simulink model "straight_forward_uniform_wind"  (R2020b)
settings: Solver=VariableStepAuto  StartTime=0.0  StopTime=10.0  RelTol=1e-3
settings Model: Creator=Dogukan  LastModifiedBy=Dogukan

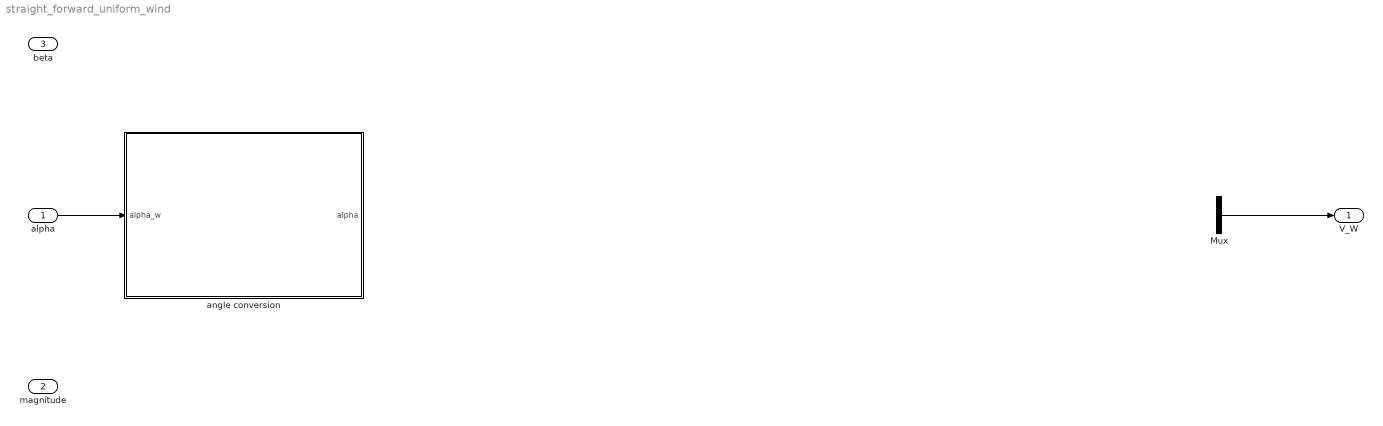
== system straight_forward_uniform_wind ==
  alpha : Inport
  magnitude : Inport  Port=2
  beta : Inport  Port=3
  Mux : Mux  Inputs=3
  angle conversion : Subsystem
  V_W : Outport
  wires:
  alpha/1 -> angle conversion/1(alpha_w)
  Mux/1 -> V_W/1

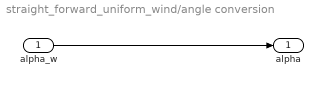
== system straight_forward_uniform_wind/angle conversion ==
  alpha_w : Inport
  alpha : Outport
  wires:
  alpha_w/1 -> alpha/1
